simulink model "Modell_13_4"  (R2018a)
settings: Solver=VariableStepAuto  StartTime=0.0  StopTime=10  RelTol=1e-3
InitFcn:
  | init_13_4
values from neighbouring files (symbols this model uses):
  a = 1    [init_13_1.m]    (also in init_13_1_v2.m; init_13_4.m)
  b = 1    [init.m]    (also in init_13_1.m; init_13_1_v2.m = 0.1111; init_13_4.m)
  kS = 1    [init_13_1_v2.m]    (also in init_13_4.m = 0.2)
  kT = 1    [init_13_1_v2.m]    (also in init_13_4.m)
  S01 = 30    [init_13_1_v2.m]    (also in init_13_4.m = 1)
  S02 = 35    [init_13_1_v2.m]    (also in init_13_4.m = 1.3)
  T01 = 29    [init_13_1_v2.m]    (also in init_13_4.m = 1.2)
  T02 = 12    [init_13_1_v2.m]    (also in init_13_4.m = 1)
libraries: simulink x6
settings Model: Creator=Uni  LastModifiedBy=Uni

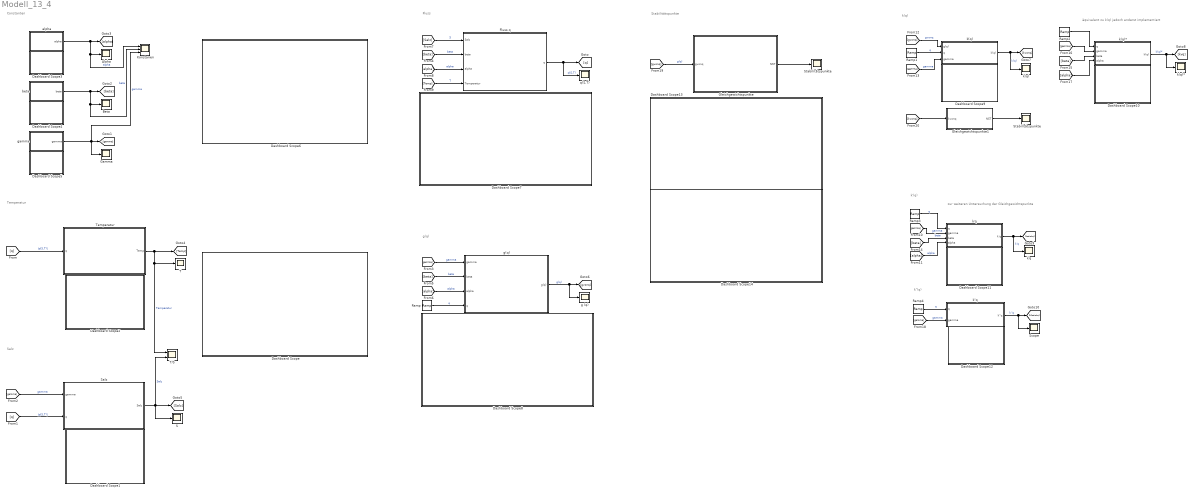
== system Modell_13_4 ==
  note: zur weiteren Untersuchung der Gleichgewichtspunkte
  note: äquivalent zu k(q) jedoch anderst implementiert
  note: Constanten
  note: Temperatur
  note: Salz
  note: Fluss
  note: g(q)
  note: k(q)
  note: k'(q)
  note: k''(q)
  note: Stabilitätspunkte
  "Alpha  " : Scope
  "Beta  " : Scope
  Dashboard Scope : Subsystem  DialogController=hmiCreateDDGDialog  IsWebBlock=on  mask(MWDashboardBlock){webBlockId=854b461d-b81b-4331-ae50-240d57b21fb6, webBlockType=sdiscope, ShowInitialText=on, HMISrcModelName=Modell_13_4}
      mask prompts: webBlockId "WebBlock Id"; webBlockType "WebBlock Type"; HMISrcModelName "Source Model"
      mask help: SimulinkHMI:dialogs:HMIScopeDialogDesc
      mask Help: helpview([docroot '/mapfiles/simulink.map'], 'hmi_scope')
      mask Display:
      | if strcmp(get_param(bdroot(gcb),'BlockDiagramType'), 'library')
      |     image([(matlabroot) '/toolbox/simulink/hmi/icons/DashboardScope.png']);
      | end
  Dashboard Scope1 : Subsystem  DialogController=hmiCreateDDGDialog  IsWebBlock=on  mask(MWDashboardBlock){webBlockId=7f7a471b-39fc-4547-a7c6-677876030e47, webBlockType=sdiscope, ShowInitialText=on, HMISrcModelName=Modell_13_4}
      mask prompts: webBlockId "WebBlock Id"; webBlockType "WebBlock Type"; HMISrcModelName "Source Model"
      mask help: SimulinkHMI:dialogs:HMIScopeDialogDesc
      mask Help: helpview([docroot '/mapfiles/simulink.map'], 'hmi_scope')
      mask Display:
      | if strcmp(get_param(bdroot(gcb),'BlockDiagramType'), 'library')
      |     image([(matlabroot) '/toolbox/simulink/hmi/icons/DashboardScope.png']);
      | end
  Dashboard Scope10 : Subsystem  DialogController=hmiCreateDDGDialog  IsWebBlock=on  mask(MWDashboardBlock){webBlockId=e9faae5f-bdb8-4bd3-b82d-94e99010152a, webBlockType=sdiscope, ShowInitialText=on, HMISrcModelName=Modell_13_4}
      mask prompts: webBlockId "WebBlock Id"; webBlockType "WebBlock Type"; HMISrcModelName "Source Model"
      mask help: SimulinkHMI:dialogs:HMIScopeDialogDesc
      mask Help: helpview([docroot '/mapfiles/simulink.map'], 'hmi_scope')
      mask Display:
      | if strcmp(get_param(bdroot(gcb),'BlockDiagramType'), 'library')
      |     image([(matlabroot) '/toolbox/simulink/hmi/icons/DashboardScope.png']);
      | end
  Dashboard Scope11 : Subsystem  DialogController=hmiCreateDDGDialog  IsWebBlock=on  mask(MWDashboardBlock){webBlockId=d754939e-ca63-44a8-967f-c9c516d626a3, webBlockType=sdiscope, ShowInitialText=on, HMISrcModelName=Modell_13_4}
      mask prompts: webBlockId "WebBlock Id"; webBlockType "WebBlock Type"; HMISrcModelName "Source Model"
      mask help: SimulinkHMI:dialogs:HMIScopeDialogDesc
      mask Help: helpview([docroot '/mapfiles/simulink.map'], 'hmi_scope')
      mask Display:
      | if strcmp(get_param(bdroot(gcb),'BlockDiagramType'), 'library')
      |     image([(matlabroot) '/toolbox/simulink/hmi/icons/DashboardScope.png']);
      | end
  Dashboard Scope12 : Subsystem  DialogController=hmiCreateDDGDialog  IsWebBlock=on  mask(MWDashboardBlock){webBlockId=49b11e21-cd19-4085-841a-4c8ad6c4669a, webBlockType=sdiscope, ShowInitialText=on, HMISrcModelName=Modell_13_4}
      mask prompts: webBlockId "WebBlock Id"; webBlockType "WebBlock Type"; HMISrcModelName "Source Model"
      mask help: SimulinkHMI:dialogs:HMIScopeDialogDesc
      mask Help: helpview([docroot '/mapfiles/simulink.map'], 'hmi_scope')
      mask Display:
      | if strcmp(get_param(bdroot(gcb),'BlockDiagramType'), 'library')
      |     image([(matlabroot) '/toolbox/simulink/hmi/icons/DashboardScope.png']);
      | end
  Dashboard Scope13 : Subsystem  DialogController=hmiCreateDDGDialog  IsWebBlock=on  mask(MWDashboardBlock){webBlockId=74d707f4-6cfa-4c83-b124-9e9615c37039, webBlockType=sdiscope, ShowInitialText=on, HMISrcModelName=Modell_13_4}
      mask prompts: webBlockId "WebBlock Id"; webBlockType "WebBlock Type"; HMISrcModelName "Source Model"
      mask help: SimulinkHMI:dialogs:HMIScopeDialogDesc
      mask Help: helpview([docroot '/mapfiles/simulink.map'], 'hmi_scope')
      mask Display:
      | if strcmp(get_param(bdroot(gcb),'BlockDiagramType'), 'library')
      |     image([(matlabroot) '/toolbox/simulink/hmi/icons/DashboardScope.png']);
      | end
  Dashboard Scope14 : Subsystem  DialogController=hmiCreateDDGDialog  IsWebBlock=on  mask(MWDashboardBlock){webBlockId=fc663eb7-b81d-4848-90d8-83969ab93d4d, webBlockType=sdiscope, ShowInitialText=on, HMISrcModelName=Modell_13_4}
      mask prompts: webBlockId "WebBlock Id"; webBlockType "WebBlock Type"; HMISrcModelName "Source Model"
      mask help: SimulinkHMI:dialogs:HMIScopeDialogDesc
      mask Help: helpview([docroot '/mapfiles/simulink.map'], 'hmi_scope')
      mask Display:
      | if strcmp(get_param(bdroot(gcb),'BlockDiagramType'), 'library')
      |     image([(matlabroot) '/toolbox/simulink/hmi/icons/DashboardScope.png']);
      | end
  Dashboard Scope2 : Subsystem  DialogController=hmiCreateDDGDialog  IsWebBlock=on  mask(MWDashboardBlock){webBlockId=1b08e5c6-2358-4da8-8eb8-13905008bf28, webBlockType=sdiscope, ShowInitialText=on, HMISrcModelName=Modell_13_4}
      mask prompts: webBlockId "WebBlock Id"; webBlockType "WebBlock Type"; HMISrcModelName "Source Model"
      mask help: SimulinkHMI:dialogs:HMIScopeDialogDesc
      mask Help: helpview([docroot '/mapfiles/simulink.map'], 'hmi_scope')
      mask Display:
      | if strcmp(get_param(bdroot(gcb),'BlockDiagramType'), 'library')
      |     image([(matlabroot) '/toolbox/simulink/hmi/icons/DashboardScope.png']);
      | end
  Dashboard Scope3 : Subsystem  DialogController=hmiCreateDDGDialog  IsWebBlock=on  mask(MWDashboardBlock){webBlockId=a47f5120-d3ce-4c5d-b3c3-8fa528aa0ec0, webBlockType=sdiscope, ShowInitialText=on, HMISrcModelName=Modell_13_4}
      mask prompts: webBlockId "WebBlock Id"; webBlockType "WebBlock Type"; HMISrcModelName "Source Model"
      mask help: SimulinkHMI:dialogs:HMIScopeDialogDesc
      mask Help: helpview([docroot '/mapfiles/simulink.map'], 'hmi_scope')
      mask Display:
      | if strcmp(get_param(bdroot(gcb),'BlockDiagramType'), 'library')
      |     image([(matlabroot) '/toolbox/simulink/hmi/icons/DashboardScope.png']);
      | end
  Dashboard Scope4 : Subsystem  DialogController=hmiCreateDDGDialog  IsWebBlock=on  mask(MWDashboardBlock){webBlockId=5cf636ce-0408-41c8-9564-e2cc551487d2, webBlockType=sdiscope, ShowInitialText=on, HMISrcModelName=Modell_13_4}
      mask prompts: webBlockId "WebBlock Id"; webBlockType "WebBlock Type"; HMISrcModelName "Source Model"
      mask help: SimulinkHMI:dialogs:HMIScopeDialogDesc
      mask Help: helpview([docroot '/mapfiles/simulink.map'], 'hmi_scope')
      mask Display:
      | if strcmp(get_param(bdroot(gcb),'BlockDiagramType'), 'library')
      |     image([(matlabroot) '/toolbox/simulink/hmi/icons/DashboardScope.png']);
      | end
  Dashboard Scope5 : Subsystem  DialogController=hmiCreateDDGDialog  IsWebBlock=on  mask(MWDashboardBlock){webBlockId=c9c44e21-7c58-423a-a168-a527239bde70, webBlockType=sdiscope, ShowInitialText=on, HMISrcModelName=Modell_13_4}
      mask prompts: webBlockId "WebBlock Id"; webBlockType "WebBlock Type"; HMISrcModelName "Source Model"
      mask help: SimulinkHMI:dialogs:HMIScopeDialogDesc
      mask Help: helpview([docroot '/mapfiles/simulink.map'], 'hmi_scope')
      mask Display:
      | if strcmp(get_param(bdroot(gcb),'BlockDiagramType'), 'library')
      |     image([(matlabroot) '/toolbox/simulink/hmi/icons/DashboardScope.png']);
      | end
  Dashboard Scope6 : Subsystem  DialogController=hmiCreateDDGDialog  IsWebBlock=on  mask(MWDashboardBlock){webBlockId=0b603d14-c2c9-4b2c-b2f2-9b03c16b8633, webBlockType=sdiscope, ShowInitialText=on, HMISrcModelName=Modell_13_4}
      mask prompts: webBlockId "WebBlock Id"; webBlockType "WebBlock Type"; HMISrcModelName "Source Model"
      mask help: SimulinkHMI:dialogs:HMIScopeDialogDesc
      mask Help: helpview([docroot '/mapfiles/simulink.map'], 'hmi_scope')
      mask Display:
      | if strcmp(get_param(bdroot(gcb),'BlockDiagramType'), 'library')
      |     image([(matlabroot) '/toolbox/simulink/hmi/icons/DashboardScope.png']);
      | end
  Dashboard Scope7 : Subsystem  DialogController=hmiCreateDDGDialog  IsWebBlock=on  mask(MWDashboardBlock){webBlockId=c70abfab-ecf9-4bec-b1b7-c632d18348ec, webBlockType=sdiscope, ShowInitialText=on, HMISrcModelName=Modell_13_4}
      mask prompts: webBlockId "WebBlock Id"; webBlockType "WebBlock Type"; HMISrcModelName "Source Model"
      mask help: SimulinkHMI:dialogs:HMIScopeDialogDesc
      mask Help: helpview([docroot '/mapfiles/simulink.map'], 'hmi_scope')
      mask Display:
      | if strcmp(get_param(bdroot(gcb),'BlockDiagramType'), 'library')
      |     image([(matlabroot) '/toolbox/simulink/hmi/icons/DashboardScope.png']);
      | end
  Dashboard Scope8 : Subsystem  DialogController=hmiCreateDDGDialog  IsWebBlock=on  mask(MWDashboardBlock){webBlockId=2b5c55f2-ffa8-44da-abc3-f3dfc5f5c374, webBlockType=sdiscope, ShowInitialText=on, HMISrcModelName=Modell_13_4}
      mask prompts: webBlockId "WebBlock Id"; webBlockType "WebBlock Type"; HMISrcModelName "Source Model"
      mask help: SimulinkHMI:dialogs:HMIScopeDialogDesc
      mask Help: helpview([docroot '/mapfiles/simulink.map'], 'hmi_scope')
      mask Display:
      | if strcmp(get_param(bdroot(gcb),'BlockDiagramType'), 'library')
      |     image([(matlabroot) '/toolbox/simulink/hmi/icons/DashboardScope.png']);
      | end
  Dashboard Scope9 : Subsystem  DialogController=hmiCreateDDGDialog  IsWebBlock=on  mask(MWDashboardBlock){webBlockId=a8edbba9-a096-42fb-b278-9aa01456f4ca, webBlockType=sdiscope, ShowInitialText=on, HMISrcModelName=Modell_13_4}
      mask prompts: webBlockId "WebBlock Id"; webBlockType "WebBlock Type"; HMISrcModelName "Source Model"
      mask help: SimulinkHMI:dialogs:HMIScopeDialogDesc
      mask Help: helpview([docroot '/mapfiles/simulink.map'], 'hmi_scope')
      mask Display:
      | if strcmp(get_param(bdroot(gcb),'BlockDiagramType'), 'library')
      |     image([(matlabroot) '/toolbox/simulink/hmi/icons/DashboardScope.png']);
      | end
  Fluss q : Subsystem
  "Gamma  " : Scope
  Gleichgewichtspunkte : Subsystem
  Gleichgewichtspunkte1 : Subsystem
  Konstanen : Scope  NumInputPorts=3
  Ramp{,1..4} (5 alike) : simulink/Sources/Ramp  slope=1  start=0  InitialOutput=0
  S : Scope
  Salz : Subsystem
  Scope : Scope
  Stabilitätspunkte : Scope
  "Stabilitätspunkte " : Scope
  T : Scope
  T/S : Scope  NumInputPorts=2
  Temperatur : Subsystem
  alpha : Subsystem
  beta : Subsystem
  g (q) : Scope
  g(q) : Subsystem
  gamma : Subsystem
  k''q : Subsystem
  k'q : Subsystem
  "k'q " : Scope
  k(q) : Subsystem
  "k(q) " : Scope
  k(q)* : Subsystem
  "k(q)* " : Scope
  q(S,T) : Scope
  wires:
  Fluss q/1(q) -> q(S,T)/1, [q]  "q(S,T)"
  gamma/1(gamma) -> Konstanen/3, "Gamma  "/1, [gamma]  "gamma"
  g(q)/1(g(q)) -> [gvonq], g (q)/1  "g(q)"
  [q] -> Salz/2(q)  "|q(S,T)|"
  [q] -> Temperatur/1(q)  "|q(S,T)|"
  [gamma] -> g(q)/1(gamma)  "gamma"
  [gamma] -> Salz/1(gamma)  "gamma"
  beta/1(beta) -> "Beta  "/1, Konstanen/2, [beta]  "beta"
  [beta] -> Fluss q/2(beta)  "beta"
  [beta] -> g(q)/2(beta)  "beta"
  alpha/1(alpha) -> "Alpha  "/1, Konstanen/1, [alpha]  "alpha"
  Temperatur/1(Temp) -> [Temp], T/1, T/S/1  "Temperatur"
  Salz/1("Salz ") -> S/1, [Salz], T/S/2  "Salz"
  [Salz] -> Fluss q/1(Salz)  "S"
  [alpha] -> Fluss q/3(alpha)  "alpha"
  [Temp] -> Fluss q/4(Temperatur)  "T"
  [gvonq] -> k(q)/1(g(q))  "gvonq"
  Ramp1/1 -> k(q)/2(q)  "q"
  [gamma] -> k(q)/3(gamma)  "gamma"
  k(q)/1(k(q)) -> "k(q) "/1, [kvonq]  "k(q)"
  k(q)*/1(k(q)) -> "k(q)* "/1, [kvq]  "k(q)*"
  [gamma] -> k(q)*/2(gamma)
  [beta] -> k(q)*/3("beta ")
  [alpha] -> k(q)*/4(alpha)
  Ramp/1 -> g(q)/4(q)  "q"
  Ramp2/1 -> k(q)*/1(q)
  Ramp3/1 -> k'q/1(q)  "q"
  [gamma] -> k'q/2(gamma)  "gamma"
  [beta] -> k'q/3(beta)  "beta"
  [alpha] -> k'q/4(alpha)  "alpha"
  k'q/1(k'q) -> "k'q "/1, [kstrichq]  "k'q"
  Ramp4/1 -> k''q/1(q)  "q"
  [gamma] -> k''q/2(gamma)  "gamma"
  k''q/1(k''q) -> Scope/1, [k2strichq]  "k''q"
  [alpha] -> g(q)/3(alpha)  "alpha"
  [gvonq] -> Gleichgewichtspunkte/1(gvonq)  "g(q)"
  Gleichgewichtspunkte/1(NST) -> Stabilitätspunkte/1
  [kvonq] -> Gleichgewichtspunkte1/1(kvonq)
  Gleichgewichtspunkte1/1(NST) -> "Stabilitätspunkte "/1

== system Modell_13_4/Dashboard Scope ==

== system Modell_13_4/Dashboard Scope1 ==

== system Modell_13_4/Dashboard Scope10 ==

== system Modell_13_4/Dashboard Scope11 ==

== system Modell_13_4/Dashboard Scope12 ==

== system Modell_13_4/Dashboard Scope13 ==

== system Modell_13_4/Dashboard Scope14 ==

== system Modell_13_4/Dashboard Scope2 ==

== system Modell_13_4/Dashboard Scope3 ==

== system Modell_13_4/Dashboard Scope4 ==

== system Modell_13_4/Dashboard Scope5 ==

== system Modell_13_4/Dashboard Scope6 ==

== system Modell_13_4/Dashboard Scope7 ==

== system Modell_13_4/Dashboard Scope8 ==

== system Modell_13_4/Dashboard Scope9 ==

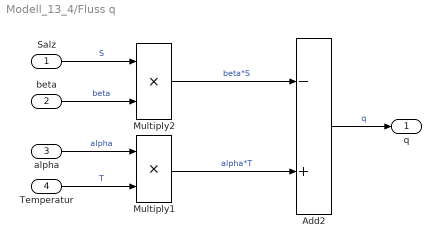
== system Modell_13_4/Fluss q ==
  Salz : Inport
  beta : Inport  Port=2
  alpha : Inport  Port=3
  Temperatur : Inport  Port=4
  Add2 : Sum  Inputs=-+
  Multiply1 : Product
  Multiply2 : Product
  q : Outport
  wires:
  Multiply2/1 -> Add2/1  "beta*S"
  beta/1 -> Multiply2/2  "beta"
  Temperatur/1 -> Multiply1/2  "T"
  Multiply1/1 -> Add2/2  "alpha*T"
  Salz/1 -> Multiply2/1  "S"
  Add2/1 -> q/1  "q"
  alpha/1 -> Multiply1/1  "alpha"

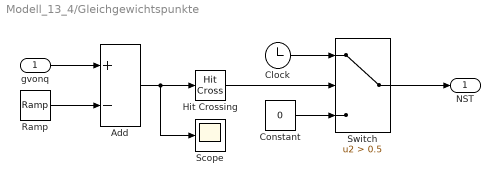
== system Modell_13_4/Gleichgewichtspunkte ==
  gvonq : Inport
  Add : Sum  Inputs=+-
  Clock : Clock
  Constant : Constant  Value=0
  Hit Crossing : HitCross
  Ramp : simulink/Sources/Ramp  slope=1  start=0  InitialOutput=0
  Scope : Scope
  Switch : Switch  Criteria=u2 > Threshold  Threshold=0.5
  NST : Outport
  wires:
  Constant/1 -> Switch/3
  Hit Crossing/1 -> Switch/2
  Switch/1 -> NST/1
  Clock/1 -> Switch/1
  gvonq/1 -> Add/1
  Add/1 -> Scope/1, Hit Crossing/1
  Ramp/1 -> Add/2

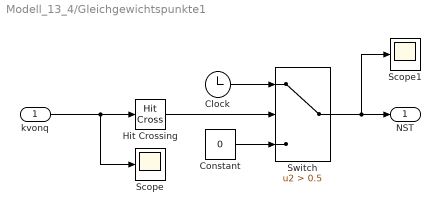
== system Modell_13_4/Gleichgewichtspunkte1 ==
  kvonq : Inport
  Clock : Clock
  Constant : Constant  Value=0
  Hit Crossing : HitCross
  Scope : Scope
  Scope1 : Scope
  Switch : Switch  Criteria=u2 > Threshold  Threshold=0.5
  NST : Outport
  wires:
  kvonq/1 -> Hit Crossing/1, Scope/1
  Clock/1 -> Switch/1
  Switch/1 -> Scope1/1, NST/1
  Hit Crossing/1 -> Switch/2
  Constant/1 -> Switch/3

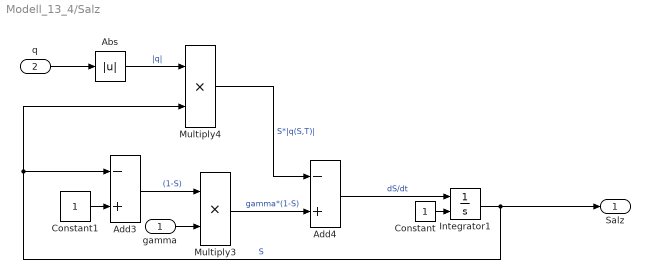
== system Modell_13_4/Salz ==
  gamma : Inport
  q : Inport  Port=2
  Abs : Abs
  Add3 : Sum  Inputs=-+
  Add4 : Sum  Inputs=-+
  Constant : Constant  VectorParams1D=off  SampleTime=-1
  Constant1 : Constant
  Integrator1 : Integrator  InitialConditionSource=external  InitialCondition=1
  Multiply3 : Product
  Multiply4 : Product
  "Salz " : Outport
  wires:
  Multiply3/1 -> Add4/2  "gamma*(1-S)"
  Integrator1/1 -> Add3/1, Multiply4/2, "Salz "/1  "S"
  Add3/1 -> Multiply3/1  "(1-S)"
  Add4/1 -> Integrator1/1  "dS/dt"
  gamma/1 -> Multiply3/2
  Multiply4/1 -> Add4/1  "S*|q(S,T)|"
  Constant1/1 -> Add3/2
  q/1 -> Abs/1
  Abs/1 -> Multiply4/1  "|q|"
  Constant/1 -> Integrator1/2

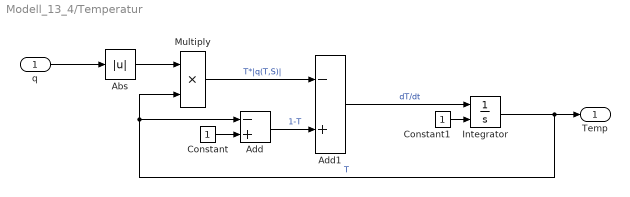
== system Modell_13_4/Temperatur ==
  q : Inport
  Abs : Abs
  Add : Sum  Inputs=-+
  Add1 : Sum  Inputs=-+
  Constant : Constant
  Constant1 : Constant
  Integrator : Integrator  InitialConditionSource=external
  Multiply : Product
  Temp : Outport
  wires:
  Integrator/1 -> Add/1, Multiply/2, Temp/1  "T"
  Add/1 -> Add1/2  "1-T"
  q/1 -> Abs/1
  Multiply/1 -> Add1/1  "T*|q(T,S)|"
  Constant/1 -> Add/2
  Add1/1 -> Integrator/1  "dT/dt"
  Constant1/1 -> Integrator/2
  Abs/1 -> Multiply/1

== system Modell_13_4/alpha ==
  (a*b)/kT : Subsystem
  Constant1 : Constant  Value=2
  Multiply4 : Product  Inputs=3
  T0star : Subsystem
  alpha : Outport
  wires:
  (a*b)/kT/1((a*b)/kT) -> Multiply4/2  "(ab)/kT"
  Multiply4/1 -> alpha/1  "alpha"
  T0star/1(T0star) -> Multiply4/3  "T0star"
  Constant1/1 -> Multiply4/1

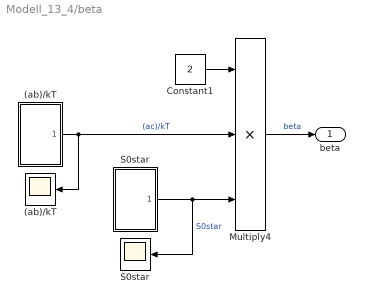
== system Modell_13_4/beta ==
  (ab)/kT : Subsystem
  "(ab)/kT " : Scope
  Constant1 : Constant  Value=2
  Multiply4 : Product  Inputs=3
  S0star : Subsystem
  "S0star " : Scope
  beta : Outport
  wires:
  Constant1/1 -> Multiply4/1
  S0star/1(S0star) -> Multiply4/3, "S0star "/1  "S0star"
  Multiply4/1 -> beta/1  "beta"
  (ab)/kT/1((a*b)/kT) -> "(ab)/kT "/1, Multiply4/2  "(ac)/kT"

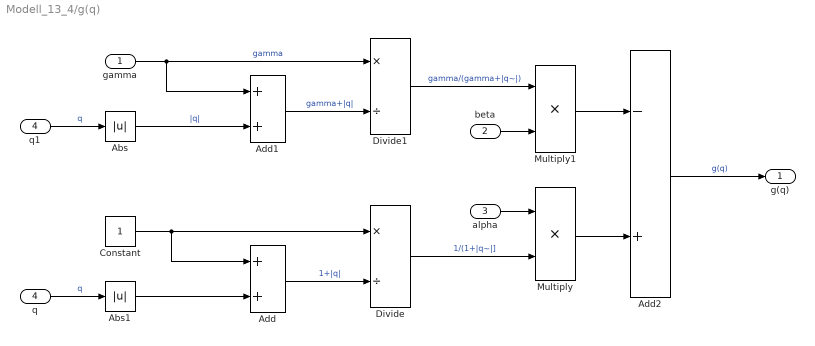
== system Modell_13_4/g(q) ==
  gamma : Inport
  beta : Inport  Port=2
  alpha : Inport  Port=3
  q : Inport  Port=4
  Abs : Abs
  Abs1 : Abs
  Add : Sum
  Add1 : Sum
  Add2 : Sum  Inputs=-+
  Constant : Constant
  Divide : Product  Inputs=*/
  Divide1 : Product  Inputs=*/
  Multiply : Product
  Multiply1 : Product
  q1 : InportShadow  Port=4
  g(q) : Outport
  wires:
  Divide1/1 -> Multiply1/1  "gamma/(gamma+|q~|)"
  Multiply/1 -> Add2/2
  Add2/1 -> g(q)/1  "g(q)"
  Add/1 -> Divide/2  "1+|q|"
  Divide/1 -> Multiply/2  "1/(1+|q~|]"
  Multiply1/1 -> Add2/1
  beta/1 -> Multiply1/2
  alpha/1 -> Multiply/1
  Constant/1 -> Add/1, Divide/1
  q/1 -> Abs1/1  "q"
  q1/1 -> Abs/1  "q"
  gamma/1 -> Add1/1, Divide1/1  "gamma"
  Add1/1 -> Divide1/2  "gamma+|q|"
  Abs/1 -> Add1/2  "|q|"
  Abs1/1 -> Add/2

== system Modell_13_4/gamma ==
  Divide : Product  Inputs=*/
  "gamma " : Scope
  kS : Constant  Value=kS
  kT : Constant  Value=kT
  gamma : Outport
  wires:
  kT/1 -> Divide/2
  kS/1 -> Divide/1
  Divide/1 -> "gamma "/1, gamma/1

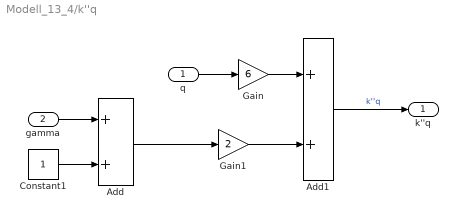
== system Modell_13_4/k''q ==
  q : Inport
  gamma : Inport  Port=2
  Add : Sum
  Add1 : Sum
  Constant1 : Constant
  Gain : Gain  Gain=6
  Gain1 : Gain  Gain=2
  k''q : Outport
  wires:
  Add1/1 -> k''q/1  "k''q"
  Gain/1 -> Add1/1
  Add/1 -> Gain1/1
  Constant1/1 -> Add/2
  Gain1/1 -> Add1/2
  gamma/1 -> Add/1
  q/1 -> Gain/1

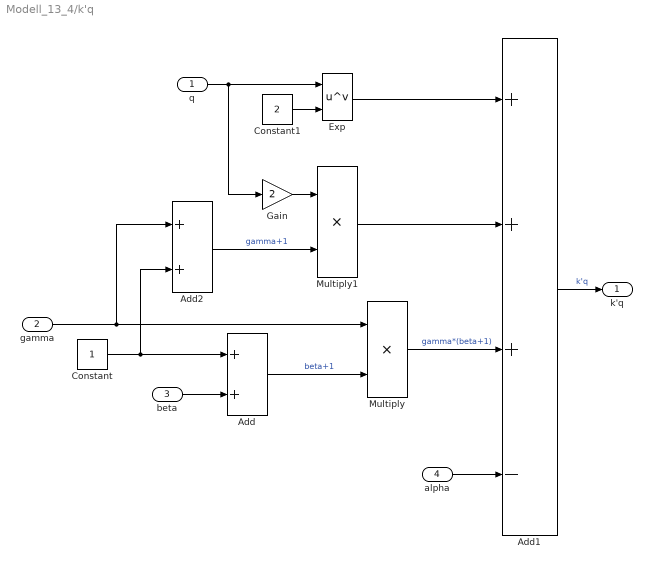
== system Modell_13_4/k'q ==
  q : Inport
  gamma : Inport  Port=2
  beta : Inport  Port=3
  alpha : Inport  Port=4
  Add : Sum
  Add1 : Sum  Inputs=+++-
  Add2 : Sum
  Constant : Constant
  Constant1 : Constant  Value=2
  Exp : Math  Operator=pow  SaturateOnIntegerOverflow=on
  Gain : Gain  Gain=2
  Multiply : Product
  Multiply1 : Product
  k'q : Outport
  wires:
  gamma/1 -> Add2/1, Multiply/1
  Constant1/1 -> Exp/2
  Constant/1 -> Add2/2, Add/1
  Exp/1 -> Add1/1
  Multiply1/1 -> Add1/2
  beta/1 -> Add/2
  Gain/1 -> Multiply1/1
  q/1 -> Gain/1, Exp/1
  Add2/1 -> Multiply1/2  "gamma+1"
  Add/1 -> Multiply/2  "beta+1"
  Multiply/1 -> Add1/3  "gamma*(beta+1)"
  Add1/1 -> k'q/1  "k'q"
  alpha/1 -> Add1/4

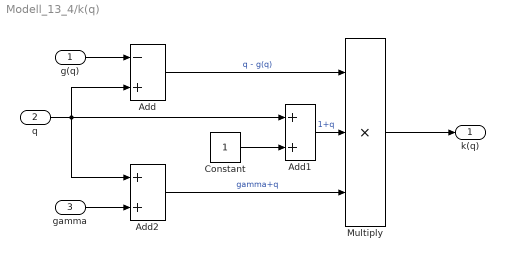
== system Modell_13_4/k(q) ==
  g(q) : Inport
  q : Inport  Port=2
  gamma : Inport  Port=3
  Add : Sum  Inputs=-+
  Add1 : Sum
  Add2 : Sum
  Constant : Constant
  Multiply : Product  Inputs=3
  k(q) : Outport
  wires:
  Add/1 -> Multiply/1  "q - g(q)"
  q/1 -> Add2/1, Add/2, Add1/1
  Multiply/1 -> k(q)/1
  gamma/1 -> Add2/2
  Add1/1 -> Multiply/2  "1+q"
  Add2/1 -> Multiply/3  "gamma+q"
  Constant/1 -> Add1/2
  g(q)/1 -> Add/1

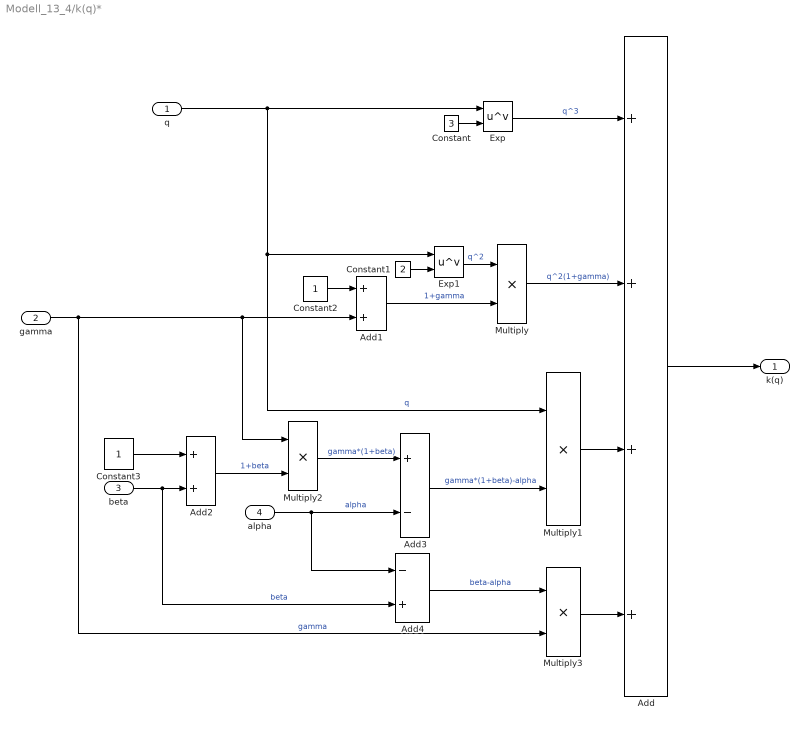
== system Modell_13_4/k(q)* ==
  q : Inport
  gamma : Inport  Port=2
  "beta " : Inport  Port=3
  alpha : Inport  Port=4
  Add : Sum  Inputs=++++
  Add1 : Sum
  Add2 : Sum
  Add3 : Sum  Inputs=+-
  Add4 : Sum  Inputs=-+
  Constant : Constant  Value=3
  Constant1 : Constant  Value=2
  Constant2 : Constant
  Constant3 : Constant
  Exp : Math  Operator=pow  SaturateOnIntegerOverflow=on
  Exp1 : Math  Operator=pow  SaturateOnIntegerOverflow=on
  Multiply{,1..3} (4 alike) : Product
  k(q) : Outport
  wires:
  q/1 -> Multiply1/1, Exp1/1, Exp/1  "q"
  Constant/1 -> Exp/2
  Exp/1 -> Add/1  "q^3"
  Constant1/1 -> Exp1/2
  Exp1/1 -> Multiply/1  "q^2"
  Constant2/1 -> Add1/1
  gamma/1 -> Multiply3/2, Multiply2/1, Add1/2  "gamma"
  Add1/1 -> Multiply/2  "1+gamma"
  Multiply/1 -> Add/2  "q^2(1+gamma)"
  Multiply1/1 -> Add/3
  "beta "/1 -> Add4/2, Add2/2  "beta"
  Constant3/1 -> Add2/1
  Add2/1 -> Multiply2/2  "1+beta"
  Multiply2/1 -> Add3/1  "gamma*(1+beta)"
  alpha/1 -> Add4/1, Add3/2  "alpha"
  Add3/1 -> Multiply1/2  "gamma*(1+beta)-alpha"
  Add4/1 -> Multiply3/1  "beta-alpha"
  Multiply3/1 -> Add/4
  Add/1 -> k(q)/1

== system Modell_13_4/alpha/(a*b)//kT ==
  Divide : Product  Inputs=*/
  Multiply3 : Product
  a : Constant  Value=a
  b : Constant  Value=b
  kT : Constant  Value=kT
  (a*b)/kT : Outport
  wires:
  b/1 -> Multiply3/2  "b"
  kT/1 -> Divide/2
  Multiply3/1 -> Divide/1  "a*b"
  Divide/1 -> (a*b)/kT/1  "(a*b)/kT"
  a/1 -> Multiply3/1  "a"

== system Modell_13_4/alpha/T0star ==
  Add3 : Sum  Inputs=+-
  T01 : Constant  Value=T01
  T02 : Constant  Value=T02
  T0star : Outport
  wires:
  T01/1 -> Add3/1
  Add3/1 -> T0star/1  "T0star"
  T02/1 -> Add3/2

== system Modell_13_4/beta/(ab)//kT ==
  Divide : Product  Inputs=*/
  Multiply3 : Product
  a : Constant  Value=a
  b : Constant  Value=b
  kT : Constant  Value=kT
  (a*b)/kT : Outport
  wires:
  a/1 -> Multiply3/1  "a"
  Divide/1 -> (a*b)/kT/1  "(a*b)/kT"
  Multiply3/1 -> Divide/1  "a*b"
  kT/1 -> Divide/2
  b/1 -> Multiply3/2  "b"

== system Modell_13_4/beta/S0star ==
  Add3 : Sum  Inputs=+-
  S01 : Constant  Value=S01
  S02 : Constant  Value=S02
  S0star : Outport
  wires:
  Add3/1 -> S0star/1  "S0star"
  S01/1 -> Add3/1
  S02/1 -> Add3/2
